simulink model "non_lin_dyn_model"  (R2024b)
settings: Solver=ode4  StartTime=0.0  StopTime=30  FixedStep=ST  RelTol=1e-3
values from neighbouring files (symbols this model uses):
  AOP = 2.75*pi/180    (= 0.0479965544298)    [parameters.m]
  AOPTR = 0    [parameters.m]
  ASLOPE = 6.28    [parameters.m]
  ASLOPETR = 6.28    [parameters.m]
  att_sp = 0    [FEL_RBFNN.m]    (also in results.m)
  Ax = 5.5*0.3048^2    (= 0.51096672)    [parameters.m]
  Ay = 156.1*0.3048^2    (= 14.502164544)    [parameters.m]
  Az = 84.7*0.3048^2    (= 7.868887488)    [parameters.m]
  B_inv = inv(B*B_dim)    [parameters.m]
  BLADES = 2    [parameters.m]
  BLADESTR = 2    [parameters.m]
  CD_mr = [0.009 0 0.3]    [parameters.m]
  CD_tr = [0.009 0 0.3]    [parameters.m]
  CHORD = 2.25*Ft_m    (= 0.6858)    [parameters.m]
  CHORDTR = 0.7*Ft_m    (= 0.21336)    [parameters.m]
  eta = 1    [FEL_RBFNN.m]
  f = [ 0; 0; Q_mr_trim/Izz]    [parameters.m]
  g = 9.81    [parameters.m]
  GAMMA = 5.216    [parameters.m]
  k = diag([3.7,5,10])    [FEL_RBFNN.m]
  k_ind = 1    [parameters.m]
  L_fus = [ -0.1 ... (first row only)    [parameters.m]
  L_mr = [  -0.1 ... (first row only)    [parameters.m]
  L_tr = [  -8.25 ... (first row only)    [parameters.m]
  lambda = diag([0.08,0.05,1.5])    [FEL_RBFNN.m]
  lat_cyc_range = [ -15 15 ]    [parameters.m]
  lon_cyc_range = [ -15 15 ]    [parameters.m]
  m = 8000*Lb_Kg    (= 3628.736)    [parameters.m]
  mr_coll_range = [ 7.5 25 ]    [parameters.m]
  NN_state = 1    [FEL_RBFNN.m]    (also in results.m)
  OMEGA = 314*(pi/30)    (= 32.8820031076)    [parameters.m]
  OMEGATR = 1608.5*(pi/30)    (= 168.44172611)    [parameters.m]
  pilot_trim = [-0.11603144404 0.198191531149 -0.14266835704 0.401015389998]    [hover_trim.mat]
  rho = 1.225    [parameters.m]
  ROTOR = 22*Ft_m    (= 6.7056)    [parameters.m]
  ROTORTR = 4.25*Ft_m    (= 1.2954)    [parameters.m]
  sigma = linspace(1.2,4.2,neurons)'    [FEL_RBFNN.m]
  ST = 0.01    [parameters.m]
  T_flap = 16/GAMMA/OMEGA    (= 0.0932876459059)    [parameters.m]
  THETT = -10*(pi/180)    (= -0.174532925199)    [parameters.m]
  THETTTR = 0*(pi/180)    (= 0)    [parameters.m]
  tr_coll_range = [ -20 20 ]    [parameters.m]
  vel_sp = 1    [FEL_RBFNN.m]    (also in results.m = 0)
  W0 = zeros(neurons,3)    [FEL_RBFNN.m]
  wind = 0    [FEL_RBFNN.m]    (also in results.m = 1)
  x0 = linspace(-1,1,neurons)'    [FEL_RBFNN.m]
  Xe_0 = [ 16404 0 -100 ]'*Ft_m    [parameters.m]
undefined symbols (not defined in the file or in its folder): rad, s
libraries: matrix_library x3, slpidlib x3, aerolibsim3d x2, sim3dlib x1, aerolibconvert2 x1, shared6dof x1, aerolibanimutils x1
(part 2 of 2)

== matlab function non_lin_dyn_model/ATTITUDE CONTROLLER/MATLAB Function1 ==
  data: time input; euler_sp output; att_sp input
function euler_sp = fcn(time,att_sp)

T = 15;

if att_sp == 2
    phi_sp   = 10*cos(2*pi*time/T-pi/3);
    theta_sp = 5*cos(2*pi*time/T-pi/3);
    psi_sp   = 0*cos(2*pi*time/T-pi/3);
elseif att_sp == 1
    phi_sp   = 10;
    theta_sp = 5;
    psi_sp   = 15;
else
    phi_sp   = 0;
    theta_sp = 0;
    psi_sp   = 0;
end

euler_sp = [phi_sp;theta_sp;psi_sp]*pi/180;

== matlab function non_lin_dyn_model/6DOF HELICOPTER/HELICOPTER FORCES AND MOMENTS/CONTROL MIXER/CYCLIC MIXING MATRIX ==
  data: mixing_matrix output
function mixing_matrix = fcn()

mixing_matrix = [1  0;
                 0 -1];

== matlab function non_lin_dyn_model/6DOF HELICOPTER/HELICOPTER FORCES AND MOMENTS/CONTROL MIXER/DIMENSIONALIZATION ==
  data: deltaA input; deltaB input; deltaC input; deltaP input; lat_cyc output; lon_cyc output; mr_coll output; tr_coll output; lat_cyc_range input; lon_cyc_range input; mr_coll_range input; tr_coll_range input
function [lat_cyc,lon_cyc,mr_coll,tr_coll] = fcn(deltaA,deltaB,deltaC,deltaP,lat_cyc_range,lon_cyc_range,mr_coll_range,tr_coll_range)

lat_cyc = (deltaA*0.5*(lat_cyc_range(2)-lat_cyc_range(1))+0.5*(lat_cyc_range(2)+lat_cyc_range(1)))*pi/180;
lon_cyc = (deltaB*0.5*(lon_cyc_range(2)-lon_cyc_range(1))+0.5*(lon_cyc_range(2)+lon_cyc_range(1)))*pi/180;
mr_coll = (deltaC*0.5*(mr_coll_range(2)-mr_coll_range(1))+0.5*(mr_coll_range(2)+mr_coll_range(1)))*pi/180;
tr_coll = (deltaP*0.5*(tr_coll_range(2)-tr_coll_range(1))+0.5*(tr_coll_range(2)+tr_coll_range(1)))*pi/180;

== matlab function non_lin_dyn_model/6DOF HELICOPTER/HELICOPTER FORCES AND MOMENTS/MAIN ROTOR/FLAPPING/INHERENT FLAPPING ==
  data: A1s input; B1s input; TAS input; a1s output; b1s output; omega input; v_i input; a_0 input; theta0_mr input; OMEGA input; ROTOR input; THETT input; GAMMA input
function [a1s,b1s] = fcn(A1s,B1s,TAS,omega,v_i,a_0,theta0_mr,OMEGA,ROTOR,THETT,GAMMA)

p = omega(1);
q = omega(2);
lambda = (-TAS(3)-v_i)/(OMEGA*ROTOR); % total inflow ratio
mu = sqrt(TAS(1)^2+TAS(2)^2)/(OMEGA*ROTOR); % rotor advance ratio in hub-wind axis
beta_w = atan2(TAS(2),TAS(1)); % rotor sideslip angle in hub-wind axis

% rotate body angular rates from hub-body to hub-wind frame:
pW = p*cos(beta_w)+q*sin(beta_w);
qW = -p*sin(beta_w)+q*cos(beta_w);

% rotate feathering angles from hub-body to hub-wind axis
A1 = A1s*cos(beta_w)-B1s*sin(beta_w);
B1 = A1s*sin(beta_w)+B1s*cos(beta_w);

% calculate wind induced flapping 
a1 = (8/3*theta0_mr*mu+2*THETT*mu-B1*(1+3/2*mu^2)-2*mu*lambda)/(1-mu^2/2) + (-16/GAMMA*qW/OMEGA + pW/OMEGA)/(1-mu^2/2);
b1 = A1+(4/3*mu*a_0)/(1+mu^2/2) + (-16/GAMMA*pW/OMEGA - qW/OMEGA)/(1+mu^2/2);

% rotate flapping angles from hub-wind to hub-body axis
a1s = a1*cos(beta_w)+b1*sin(beta_w);
b1s = -a1*sin(beta_w)+b1*cos(beta_w);

== matlab function non_lin_dyn_model/6DOF HELICOPTER/HELICOPTER FORCES AND MOMENTS/MAIN ROTOR/FLAPPING/flapping restraint ==
  data: max_flap input; a1s output; b1s output; a0 input; stop output; a1s input; b1s input
function [a1s,b1s,stop] = fcn(max_flap,a0,a1s,b1s)

beta_max = a0 + sqrt(a1s^2+b1s^2);
beta_min = a0 - sqrt(a1s^2+b1s^2);

if abs(beta_max)>max_flap ||  abs(beta_min)>max_flap
    
    %k = max_flap/(abs(a0)+sqrt(a1^2+b1^2)); %scaling factor
    k = sqrt((max_flap-abs(a0))^2)/sqrt(a1s^2+b1s^2); %scaling factor (coning unaltered)
    %a = k*[ a0 a1 b1 ]';
    a = [ a0 k*a1s k*b1s ]';
    fprintf('<strong> WARNING: main rotor blade flapping exceeded limits </strong> \n')
    stop = true;
else
    a = [ a0 a1s b1s ]';
    stop = false;
end

a1s = a(2);
b1s = a(3);

== matlab function non_lin_dyn_model/ATTITUDE CONTROLLER/ANGULAR RATE FEL CONTROLLER /CONTROL LAW ==
  data: f input; u output; B_inv input; DELTA input; s input; e input; x_sp_dot input; lambda input; k input
function u = fcn(f,B_inv,DELTA,s,e,x_sp_dot,lambda,k)


u = B_inv*(-f-DELTA+x_sp_dot-lambda*e-k*s);
